simulink subsystem "ALU"  (R2024b)
settings: Solver=VariableStepAuto  StartTime=0.0  StopTime=10.0  RelTol=1e-3
libraries: simulink x3
settings Model: Creator=stefano  LastModifiedBy=stefano
settings RTWCC: GPUComputeCapability=3.5

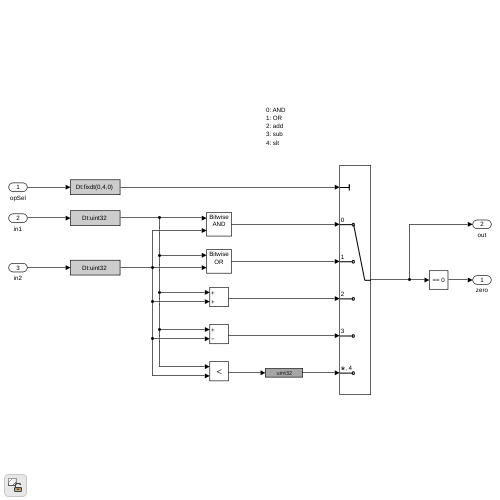
[thumbnail: Simulink's stored preview of the top-level diagram]
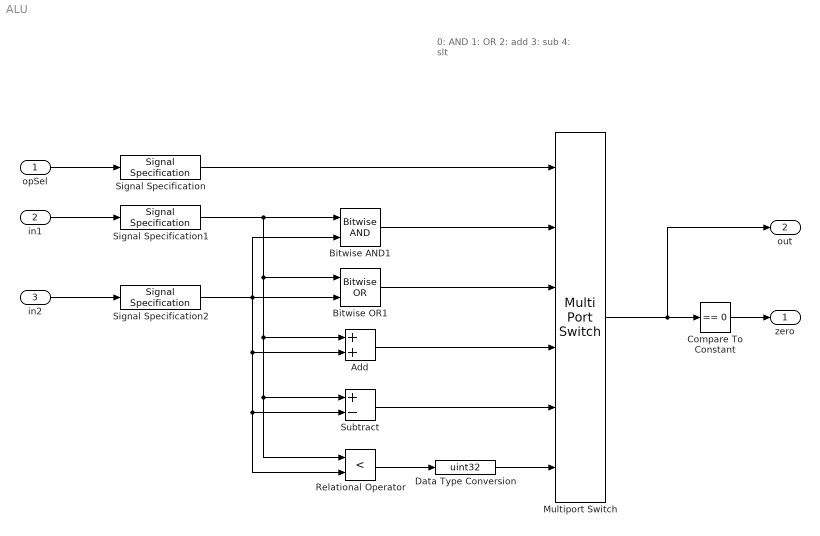
== system ALU ==
  note: 0: AND
      | 1: OR
      | 2: add
      | 3: sub
      | 4: slt
  opSel : Inport
  in1 : Inport  Port=2
  in2 : Inport  Port=3
  Add : Sum
  Bitwise AND1 : simulink/Logic and Bit Operations/Bitwise Operator  logicop=AND  UseBitMask=off  NumInputPorts=2  BitMask=bin2dec('11011001')  BitMaskRealWorld=Stored Integer
      settings: LibrarySourceBlock=|
      | simulink/Quick Insert/Logic and Bit
      | Operations/Bitwise AND
  Bitwise OR1 : simulink/Logic and Bit Operations/Bitwise Operator  logicop=OR  UseBitMask=off  NumInputPorts=2  BitMask=bin2dec('11011001')  BitMaskRealWorld=Stored Integer
      settings: LibrarySourceBlock=|
      | simulink/Quick Insert/Logic and Bit
      | Operations/Bitwise OR
  Compare To Constant : simulink/Logic and Bit Operations/Compare To Constant  relop===  const=0  OutDataTypeStr=boolean
  Data Type Conversion : DataTypeConversion  OutDataTypeStr=uint32  SaturateOnIntegerOverflow=off  RndMeth=Floor
  Multiport Switch : MultiPortSwitch  DataPortOrder=Zero-based contiguous  Inputs=5  DiagnosticForDefault=Warning  zeroidx=on  SaturateOnIntegerOverflow=off  InputSameDT=off
  Relational Operator : RelationalOperator  Operator=<  OutDataTypeStr=boolean  RndMeth=Simplest  InputSameDT=off
  Signal Specification : SignalSpecification  OutDataTypeStr=fixdt(0,4,0)
  Signal Specification1 : SignalSpecification  OutDataTypeStr=uint32
  Signal Specification2 : SignalSpecification  OutDataTypeStr=uint32
  Subtract : Sum  Inputs=+-
  zero : Outport
  out : Outport  Port=2
  wires:
  Compare To Constant/1 -> zero/1
  opSel/1 -> Signal Specification/1
  in1/1 -> Signal Specification1/1
  in2/1 -> Signal Specification2/1
  Signal Specification1/1 -> Subtract/1, Relational Operator/1, Add/1, Bitwise OR1/1, Bitwise AND1/1
  Signal Specification2/1 -> Add/2, Relational Operator/2, Subtract/2, Bitwise OR1/2, Bitwise AND1/2
  Multiport Switch/1 -> out/1, Compare To Constant/1
  Signal Specification/1 -> Multiport Switch/1
  Bitwise AND1/1 -> Multiport Switch/2
  Bitwise OR1/1 -> Multiport Switch/3
  Add/1 -> Multiport Switch/4
  Subtract/1 -> Multiport Switch/5
  Relational Operator/1 -> Data Type Conversion/1
  Data Type Conversion/1 -> Multiport Switch/6
